simulink model "ODEfunction"  (R2016a)
settings: Solver=VariableStepAuto  StartTime=0.0  StopTime=25  RelTol=1e-3
settings Model: Creator=witkey721  LastModifiedBy=witkey721

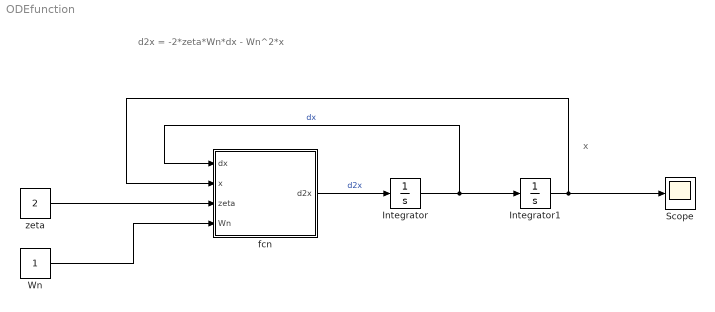
== system ODEfunction ==
  note: x
  note: d2x = -2*zeta*Wn*dx - Wn^2*x
  Integrator : Integrator
  Integrator1 : Integrator  InitialCondition=5
  Scope : Scope
  Wn : Constant
  "fcn " : MATLAB Function  TreatAsAtomicUnit=on
  zeta : Constant  Value=2
  wires:
  "fcn "/1(d2x) -> Integrator/1  "d2x"
  Integrator/1 -> "fcn "/1(dx), Integrator1/1  "dx"
  Integrator1/1 -> "fcn "/2(x), Scope/1
  zeta/1 -> "fcn "/3(zeta)
  Wn/1 -> "fcn "/4(Wn)

== matlab function ODEfunction/fcn  ==
  data: dx input; d2x output; x input; zeta input; Wn input
function d2x = fcn(dx,x,zeta,Wn)
%#codegen
d2x = -2*zeta*Wn*dx - Wn^2*x;
